simulink model "EnvironmentModel"  (R2014a)
settings: Solver=FixedStepDiscrete  StartTime=0.0  StopTime=SimLength  FixedStep=SampleTime  RelTol=1e-3
PreLoadFcn:
  | set_global_callback;
settings Model: Creator=georg  LastModifiedBy=georg

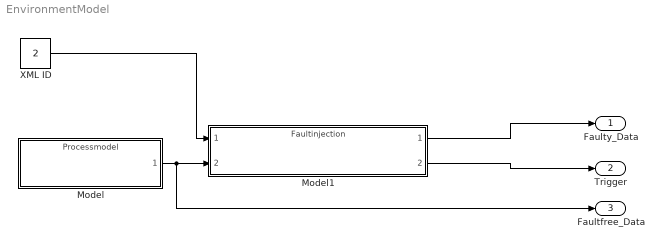
== system EnvironmentModel ==
  Model : ModelReference  ModelNameDialog=Processmodel.slx  SimulationMode=Normal  ModelReferenceVersion=1.12  CopyOfModelName=Processmodel.slx  DefaultDataLogging=on
  Model1 : ModelReference  ModelNameDialog=Faultinjection.slx  SimulationMode=Normal  ModelReferenceVersion=1.10  CopyOfModelName=Faultinjection.slx  DefaultDataLogging=on
  XML ID : Constant  Value=2  OutDataTypeStr=single
  Faulty_Data : Outport
  Trigger : Outport  Port=2
  Faultfree_Data : Outport  Port=3
  wires:
  Model/1 -> Faultfree_Data/1, Model1/2
  Model1/1 -> Faulty_Data/1
  XML ID/1 -> Model1/1
  Model1/2 -> Trigger/1
